simulink library "librairie"  (Simulink 9.0)
settings: Solver=VariableStepAuto  StartTime=0.0  StopTime=10.0  RelTol=1e-3
libraries: cstblocks x3
settings Model: Creator=DEHAEZE  LastModifiedBy=DEHAEZE

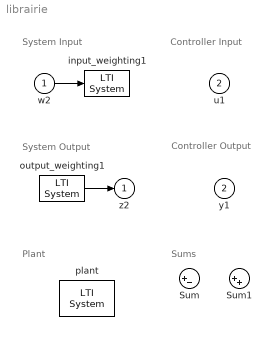
== system librairie ==
  note: Controller Input
  note: Controller Output
  note: System Input
  note: System Output
  note: Sums
  note: Plant
  w2 : Inport
  u1 : Inport  Port=2
  Sum : Sum  Inputs=|+-  SaturateOnIntegerOverflow=on  InputSameDT=on  OutDataTypeStr=Inherit: Same as first input
  Sum1 : Sum  Inputs=|++  SaturateOnIntegerOverflow=on  InputSameDT=on  OutDataTypeStr=Inherit: Same as first input
  input_weighting1 : cstblocks/LTI System  sys=W4  IC=[]
  output_weighting1 : cstblocks/LTI System  sys=W1  IC=[]
  plant : cstblocks/LTI System  sys=tf(1)  IC=[]
  z2 : Outport  InitialOutput=0
  y1 : Outport  Port=2  InitialOutput=0
  wires:
  output_weighting1/1 -> z2/1
  w2/1 -> input_weighting1/1
